simulink model "ICN_with_BR_input_model4test_clusterParams_ParkFig2C_VlungNLR"  (R2020b)
settings: Solver=ode15s  StartTime=0.5  StopTime=480  RelTol=1e-3  EnableMultiTasking=on
model workspace (MAT data in the model file):
  HRResponseIano = [1 0.976355617701 1.05061592575 1.14391807051 1.22959062218 1.30026078221 1.35513299833 1.39551709306 1.423380234 1.44057518669 1.44870724956 1.44945189675 ... (1201 elements, 1x1201)]
values from neighbouring files (symbols this model uses):
  delta_BR = Simulink.Parameter(delta_BR)    [BRclosedLoop_model_initialize_params.m]
  delta_CP = Simulink.Parameter(delta_CP)    [BRclosedLoop_model_initialize_params.m]
  delta_LS = Simulink.Parameter(delta_LS)    [BRclosedLoop_model_initialize_params.m]
  fac0 = 10    [BR_ctrl_params_LBNP_2001.m]    (also in BRmodel_ctrls_LBNP_2001.mat)
  Gal = 23.29    [BR_ctrl_params_LBNP_2001.m]    (also in BRmodel_ctrls_LBNP_2001.mat)
  kBR = Simulink.Parameter(kBR)    [BRclosedLoop_model_initialize_params.m]
  kCP = Simulink.Parameter(kCP)    [BRclosedLoop_model_initialize_params.m]
  kLS = Simulink.Parameter(kLS)    [BRclosedLoop_model_initialize_params.m]
  LBNP_input = Simulink.Parameter(LBNP_input)    [BRclosedLoop_model_initialize_params.m]
  midptCP_gain = Simulink.Parameter(midptCP_gain)    [BRclosedLoop_model_initialize_params.m]
  midptLS_gain = Simulink.Parameter(midptLS_gain)    [BRclosedLoop_model_initialize_params.m]
  minval_BR = Simulink.Parameter(minval_BR)    [BRclosedLoop_model_initialize_params.m]
  minval_CP = Simulink.Parameter(minval_CP)    [BRclosedLoop_model_initialize_params.m]
  minval_LS = Simulink.Parameter(minval_LS)    [BRclosedLoop_model_initialize_params.m]
libraries: simulink x1
(part 2 of 2)

== system ICN_with_BR_input_model4test_clusterParams_ParkFig2C_VlungNLR/Autonomic Nervous System/Emaxlv_inv ==
  fev : Inport
  fes : Inport  Port=2
  Add1 : Sum  Inputs=+++
  Add2 : Sum
  Clock : Clock
  Emaxlv0_denervated (Emaxlv0) : Constant  Value=0.25659999999999994
  Emaxlv_symp : Subsystem
  Emaxlv_vag : Subsystem
  Math Function7 : Math  Operator=reciprocal  SignedPower=on  SaturateOnIntegerOverflow=on
  Pcs_start : Constant
  Scope6 : Scope
  const : Constant  Value=0
  tstall : Switch  Criteria=u2 > Threshold  Threshold=1
  Emaxlv : Outport
  wires:
  Emaxlv_symp/1(1/Emaxlv) -> Scope6/1, Add1/2
  Math Function7/1 -> Add2/1
  Emaxlv_vag/1(1/Emaxlv) -> Add1/1
  Emaxlv0_denervated (Emaxlv0)/1 -> Add2/2
  const/1 -> Add1/3
  Clock/1 -> tstall/2
  Pcs_start/1 -> tstall/3
  tstall/1 -> Math Function7/1
  Add1/1 -> tstall/1
  fes/1 -> Emaxlv_symp/1(fes)
  fev/1 -> Emaxlv_vag/1(fev)
  Add2/1 -> Emaxlv/1

== system ICN_with_BR_input_model4test_clusterParams_ParkFig2C_VlungNLR/Autonomic Nervous System/Emaxrv_inv ==
  fev : Inport
  fes : Inport  Port=2
  Add3 : Sum  Inputs=+++
  Add4 : Sum
  Clock2 : Clock
  Emaxlv0_denervated1 : Constant  Value=1.283*0.5903
  Emaxlv_symp1 : Subsystem
  Emaxlv_vag1 : Subsystem
  Math Function2 : Math  Operator=reciprocal  SignedPower=on  SaturateOnIntegerOverflow=on
  Pcs_start2 : Constant
  Switch2 : Switch  Criteria=u2 > Threshold  Threshold=1
  const1 : Constant  Value=0
  Emaxrv : Outport
  wires:
  Switch2/1 -> Math Function2/1
  Clock2/1 -> Switch2/2
  Add3/1 -> Switch2/1
  Emaxlv_symp1/1(1/Emarlv) -> Add3/2
  Math Function2/1 -> Add4/1
  const1/1 -> Add3/3
  Emaxlv0_denervated1/1 -> Add4/2
  Pcs_start2/1 -> Switch2/3
  Emaxlv_vag1/1(1/Emaxrv) -> Add3/1
  fev/1 -> Emaxlv_vag1/1(fev)
  fes/1 -> Emaxlv_symp1/1(fes)
  Add4/1 -> Emaxrv/1

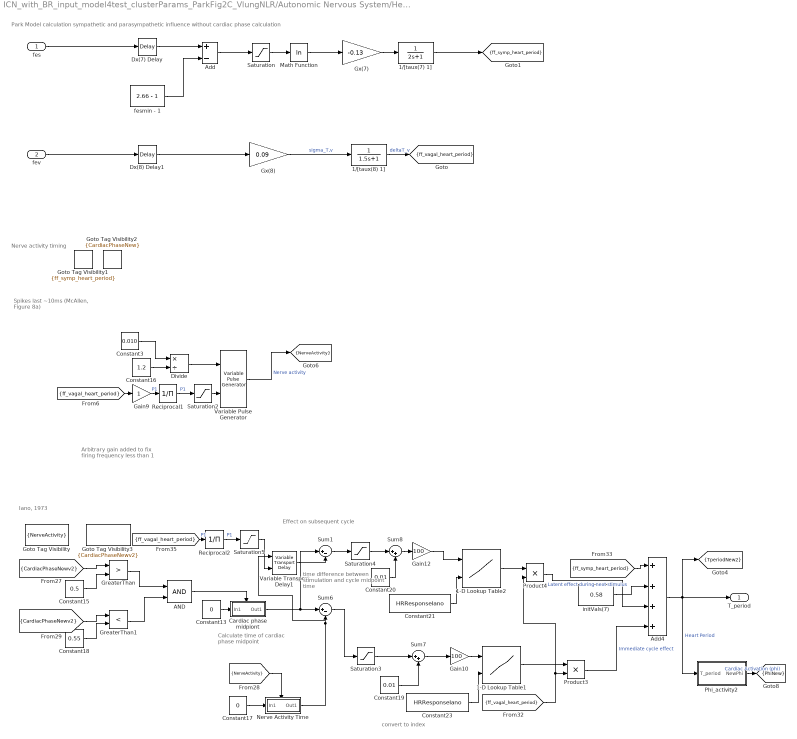
== system ICN_with_BR_input_model4test_clusterParams_ParkFig2C_VlungNLR/Autonomic Nervous System/Heart_period ==
  note: Park Model calculation sympathetic and parasympathetic influence without cardiac phase calculation
  note: Nerve activity timing
  note: convert to index
  note: time difference between stimulation and cycle midpoint time
  note: Calculate time of cardiac phase midpoint
  note: Iano, 1973
  note: Spikes last ~10ms (McAllen, Figure 8a)
  note: Arbitrary gain added to fix firing frequency less than 1
  note: Effect on subsequent cycle
  fes : Inport
  fev : Inport  Port=2
  1-D Lookup Table1 : Lookup_n-D  NumberOfTableDimensions=1  BreakpointsForDimension1=[0:1200]  BreakpointsForDimension2=[0:1199]  TableSource=Input port  Table=tanh([-5:5])  InternalRulePriority=Speed  RndMeth=Simplest  InputSameDT=on
      settings: InputPortMap=u0,p221
  1-D Lookup Table2 : Lookup_n-D  NumberOfTableDimensions=1  BreakpointsForDimension1=[0:1200]  BreakpointsForDimension2=[0:1199]  TableSource=Input port  Table=tanh([-5:5])  InternalRulePriority=Speed  RndMeth=Simplest  InputSameDT=on
      settings: InputPortMap=u0,p221
  1/[taux(7) 1] : TransferFcn  Denominator=[2 1]
  1/[taux(8) 1] : TransferFcn  Denominator=[1.5 1]
  AND : Logic  IconShape=distinctive  AllPortsSameDT=off  OutDataTypeStr=boolean
  Add : Sum  Inputs=+-
  Add4 : Sum  Inputs=++++
  Cardiac phase midpiont : Subsystem  TreatAsAtomicUnit=on
  Constant13 : Constant  Value=0
  Constant15 : Constant  Value=0.5
  Constant16 : Constant  Value=1.2
  Constant17 : Constant  Value=0
  Constant18 : Constant  Value=0.55
  Constant19 : Constant  Value=0.01
  Constant20 : Constant  Value=0.01
  Constant21 : Constant  Value=HRResponseIano
  Constant23 : Constant  Value=HRResponseIano
  Constant3 : Constant  Value=0.010
  Divide : Product  Inputs=*/
  Dx(7) Delay : TransportDelay  DelayTime=2  BufferSize=2048
  Dx(8) Delay1 : TransportDelay  DelayTime=0.2  BufferSize=2048
  Gain10 : Gain  Gain=100
  Gain12 : Gain  Gain=100
  Gain9 : Gain
  Goto Tag Visibility : GotoTagVisibility  GotoTag=NerveActivity
  Goto Tag Visibility1 : GotoTagVisibility  GotoTag=ff_symp_heart_period
  Goto Tag Visibility2 : GotoTagVisibility  GotoTag=CardiacPhaseNew
  Goto Tag Visibility3 : GotoTagVisibility  GotoTag=CardiacPhaseNewv2
  GreaterThan : RelationalOperator  Operator=>  OutDataTypeStr=boolean  RndMeth=Simplest
  GreaterThan1 : RelationalOperator  Operator=<  OutDataTypeStr=boolean  RndMeth=Simplest
  Gx(7) : Gain  Gain=-0.13
  Gx(8) : Gain  Gain=0.09
  Math Function : Math  Operator=log  SignedPower=on  SaturateOnIntegerOverflow=on
  Nerve Activity Time : Subsystem  TreatAsAtomicUnit=on
  Phi_activity2 : Subsystem
  Product3 : Product
  Product4 : Product
  Reciprocal1 : Product  Inputs=/
  Reciprocal2 : Product  Inputs=/
  Saturation : Saturate  UpperLimit=inf  LowerLimit=1
  Saturation2 : Saturate  UpperLimit=10
  Saturation3 : Saturate  UpperLimit=inf  LowerLimit=0
  Saturation4 : Saturate  UpperLimit=inf  LowerLimit=0
  Saturation5 : Saturate  UpperLimit=10
  Sum1 : Sum  Inputs=|+-
  Sum6 : Sum  Inputs=|+-
  Sum7 : Sum  Inputs=|++
  Sum8 : Sum  Inputs=|++
  Variable Transport Delay1 : VariableTransportDelay  VariableDelayType=Variable transport delay  MaximumDelay=10  MaximumPoints=2048
  Variable Pulse Generator : VariablePulseGenerator  AllowZeroPulseWidth=on  SampleTime=0.1
  fesmin - 1 : Constant  Value=2.66 - 1
  initVals(7) : Constant  Value=0.58
  T_period : Outport
  tag scope: NerveActivity=scoped, PhiNew=scoped, TperiodNew2=scoped, ff_symp_heart_period=scoped, ff_vagal_heart_period=scoped
  wires:
  Dx(7) Delay/1 -> Add/1
  fesmin - 1/1 -> Add/2
  Add/1 -> Saturation/1
  Saturation/1 -> Math Function/1
  Math Function/1 -> Gx(7)/1
  Gx(7)/1 -> 1/[taux(7) 1]/1
  fes/1 -> Dx(7) Delay/1
  fev/1 -> Dx(8) Delay1/1
  Dx(8) Delay1/1 -> Gx(8)/1
  Gx(8)/1 -> 1/[taux(8) 1]/1  "sigma_T,v"
  1/[taux(7) 1]/1 -> [ff_symp_heart_period]
  1/[taux(8) 1]/1 -> [ff_vagal_heart_period]  "deltaT_v"
  Constant3/1 -> Divide/1
  Divide/1 -> Variable Pulse Generator/1
  Constant16/1 -> Divide/2
  Variable Pulse Generator/1 -> [NerveActivity]  "Nerve activity"
  Gain9/1 -> Reciprocal1/1  "P1"
  [ff_vagal_heart_period] -> Gain9/1
  Reciprocal1/1 -> Saturation2/1  "P1"
  Saturation2/1 -> Variable Pulse Generator/2
  1-D Lookup Table1/1 -> Product3/1
  Constant13/1 -> Cardiac phase midpiont/1(In1)
  [NerveActivity] -> Nerve Activity Time/Trigger
  Constant17/1 -> Nerve Activity Time/1(In1)
  Nerve Activity Time/1(Out1) -> Variable Transport Delay1/1, Sum6/2
  [CardiacPhaseNewv2] -> GreaterThan/1
  Constant15/1 -> GreaterThan/2
  Constant18/1 -> GreaterThan1/2
  [CardiacPhaseNewv2] -> GreaterThan1/1
  GreaterThan/1 -> AND/1
  GreaterThan1/1 -> AND/2
  AND/1 -> Cardiac phase midpiont/Trigger
  Constant19/1 -> Sum7/2
  Gain10/1 -> 1-D Lookup Table1/1
  Sum7/1 -> Gain10/1
  Saturation3/1 -> Sum7/1
  Sum6/1 -> Saturation3/1
  Add4/1 -> T_period/1, [TperiodNew2], Phi_activity2/1(T_period)  "Heart Period"
  [ff_symp_heart_period] -> Add4/1
  initVals(7)/1 -> Add4/2
  Cardiac phase midpiont/1(Out1) -> Sum1/1, Sum6/1
  Sum1/1 -> Saturation4/1
  Saturation4/1 -> Sum8/1
  Constant20/1 -> Sum8/2
  Sum8/1 -> Gain12/1
  Gain12/1 -> 1-D Lookup Table2/1
  Constant21/1 -> 1-D Lookup Table2/2
  1-D Lookup Table2/1 -> Product4/1
  Product4/1 -> Add4/3  "Latent effect during next stimulus"
  [ff_vagal_heart_period] -> Product4/2, Product3/2
  Variable Transport Delay1/1 -> Sum1/2
  Saturation5/1 -> Variable Transport Delay1/2
  [ff_vagal_heart_period] -> Reciprocal2/1  "P1"
  Reciprocal2/1 -> Saturation5/1  "P1"
  Constant23/1 -> 1-D Lookup Table1/2
  Product3/1 -> Add4/4  "Immediate cycle effect"
  Phi_activity2/1(NewPhi) -> [PhiNew]  "Cardiac Activation (phi)"

== system ICN_with_BR_input_model4test_clusterParams_ParkFig2C_VlungNLR/Autonomic Nervous System/ICN ==
  note: ICN
  note: Scoped Variables
  note: Assumptions
      | Inputs to PN can be modeled as linear combinations (Shinohara, 2012; Magosso, "Theoretical analysis...connection", 2002; Park, 2020)
      | Inputs to LCN can be modeled as linear combinations with sympathetic inputs decreasing firing frequency (negative gain)
      | Only one set of LCNs (same LCN firing frequency goes to the DMV and NA principal neruons)
  fesh : Inport
  fevHR : Inport  Port=2
  fevEmax : Inport  Port=3
  fabr : Inport  Port=4
  Goto Tag Visibility1 : GotoTagVisibility  GotoTag=HR_ICN
  Goto Tag Visibility2 : GotoTagVisibility  GotoTag=phi_ICN
  Goto Tag Visibility3 : GotoTagVisibility  GotoTag=Emaxlv_ICN
  LCN : Subsystem
  PN-DMV : Subsystem
      settings: PortSchema="{\"entries\":[{\"content\":{\"sides\":[{\"content\":{\"connectorIds\":[\"In1\"]},\"type\":\"ConnectorPlacement.EquallySpacedRectSide\",\"uuid\":\"d579c9fc-b45a-4a3f-b69c-1a8b140cd445\"},{\"content\":{\"connectorIds\":[\"Out1\"],\"side\":\"RIGHT\"},\"type\":\"ConnectorPlacement.EquallySpacedRectSide\",\"uuid\":\"0e605ac8-446d-4e1b-b0e5-7b9f562202d0\"},{\"content\":{\"connectorIds\":[\"In2\"],\"side\":\"TOP\"},\"type\":\"ConnectorPlacement.EquallySpacedRectSide\",\"uuid\":\"2307843b-ee9d-4abf-8a00-d07f8ff12bca\"},{\"content\":{\"connectorIds\":[],\"side\":\"HIDDEN\"},\"type\":\"ConnectorPlacement.EquallySpacedRectSide\",\"uuid\":\"4680f609-716a-4cbc-b0ab-b941df6990b7\"}]},\"type\":\"ConnectorPlacement.EquallySpacedConnector\",\"uuid\":\"a97b8c04-f8fb-4ce5-9bdc-b62bd80eb510\"}],\"packageUris\":[\"http://schema.mathworks.com/mf0/Connector/R2020b\"],\"version\":\"1.0\"}"
  PN-NA : Subsystem
      settings: PortSchema="{\"entries\":[{\"content\":{\"sides\":[{\"content\":{\"connectorIds\":[\"In1\"]},\"type\":\"ConnectorPlacement.EquallySpacedRectSide\",\"uuid\":\"d579c9fc-b45a-4a3f-b69c-1a8b140cd445\"},{\"content\":{\"connectorIds\":[\"Out1\"],\"side\":\"RIGHT\"},\"type\":\"ConnectorPlacement.EquallySpacedRectSide\",\"uuid\":\"0e605ac8-446d-4e1b-b0e5-7b9f562202d0\"},{\"content\":{\"connectorIds\":[],\"side\":\"TOP\"},\"type\":\"ConnectorPlacement.EquallySpacedRectSide\",\"uuid\":\"2307843b-ee9d-4abf-8a00-d07f8ff12bca\"},{\"content\":{\"connectorIds\":[\"In2\"],\"side\":\"BOTTOM\"},\"type\":\"ConnectorPlacement.EquallySpacedRectSide\",\"uuid\":\"5095c59b-788d-467d-b9ae-5586250fef9c\"},{\"content\":{\"connectorIds\":[],\"side\":\"HIDDEN\"},\"type\":\"ConnectorPlacement.EquallySpacedRectSide\",\"uuid\":\"4680f609-716a-4cbc-b0ab-b941df6990b7\"}]},\"type\":\"ConnectorPlacement.EquallySpacedConnector\",\"uuid\":\"a97b8c04-f8fb-4ce5-9bdc-b62bd80eb510\"}],\"packageUris\":[\"http://schema.mathworks.com/mf0/Connector/R2020b\"],\"version\":\"1.0\"}"
  Scope : Scope  NumInputPorts=2
  To Workspace1 : ToWorkspace  VariableName=PN_DMV_ff  SampleTime=-1
  To Workspace13 : ToWorkspace  VariableName=PN_NA_ff  SampleTime=-1
  To Workspace2 : ToWorkspace  VariableName=LCN_ff  SampleTime=-1
  kBR_ICN : Gain
  fevHR_ICN : Outport
  fevEmax_ICN : Outport  Port=2
  tag scope: fev_ICN_DMV=scoped
  wires:
  kBR_ICN/1 -> LCN/3(In2)  "Afferent inputs"
  fevEmax/1 -> Scope/1, PN-DMV/1(from DMV), LCN/2(fevEmax)  "DMV output"
  fevHR/1 -> PN-NA/1(fevHR)  "NA output"
  fesh/1 -> LCN/1(fesh)  "fesh"
  PN-DMV/1(x4) -> To Workspace1/1, fevEmax_ICN/1, [fev_ICN_DMV]  "fevEmax_ICN"
  fabr/1 -> kBR_ICN/1
  PN-NA/1(Out1) -> To Workspace13/1, fevHR_ICN/1  "fevHR_ICN"
  LCN/1("from LCN ") -> PN-NA/2("from LCN "), To Workspace2/1, Scope/2, PN-DMV/2("from LCN ")  "LCN Output"

== system ICN_with_BR_input_model4test_clusterParams_ParkFig2C_VlungNLR/Autonomic Nervous System/Left ventricle ==
  Phi : Inport
  Add1 : Sum  Inputs=+-
  Add2 : Sum  Inputs=-+
  Add3 : Sum
  Constant2 : Constant
  Constant4 : Constant
  Math Function : Math  SignedPower=on  SaturateOnIntegerOverflow=on
  P0lv : Constant  Value=0.92999999999999994
  Product : Product  Inputs=3
  Product1 : Product
  Product2 : Product  Inputs=3
  Subsystem : Subsystem
  Vulv : Constant  Value=30.856799999999996
  kElv : Constant  Value=0.01638
  Pmaxlv : Outport
  wires:
  Subsystem/1(Out1) -> Product/3
  [Emaxlv] -> Product/2
  Phi/1 -> Add2/1, Product/1
  Vulv/1 -> Subsystem/1(Vulv)
  [Vlv] -> Product1/1, Subsystem/2(Vlv)
  kElv/1 -> Product1/2
  Product1/1 -> Math Function/1
  Math Function/1 -> Add1/1
  Constant2/1 -> Add1/2
  Add1/1 -> Product2/1
  P0lv/1 -> Product2/2
  Constant4/1 -> Add2/2
  Add2/1 -> Product2/3
  Product/1 -> Add3/1
  Product2/1 -> Add3/2
  Add3/1 -> Pmaxlv/1

== system ICN_with_BR_input_model4test_clusterParams_ParkFig2C_VlungNLR/Autonomic Nervous System/Lung stretch receptors ==
  Vlungs : Inport
  (1)/(tau_lung 1) : TransferFcn  Denominator=[2 1]
  Gal : Gain  Gain=23.29
  falr : Outport
  wires:
  Vlungs/1 -> Gal/1
  (1)/(tau_lung 1)/1 -> falr/1  "fal"
  Gal/1 -> (1)/(tau_lung 1)/1

== system ICN_with_BR_input_model4test_clusterParams_ParkFig2C_VlungNLR/Autonomic Nervous System/Rep ==
  fesp : Inport
  " (1)/([taux(4) 1])" : TransferFcn  Denominator=[6 1]
  Add : Sum  Inputs=+-
  Add1 : Sum
  Constant : Constant  Value=2.66 - 1
  Dx(4) Delay : TransportDelay  DelayTime=2  BufferSize=2048
  Gx(4) : Gain  Gain=0.653
  Math Function : Math  Operator=log  SignedPower=on  SaturateOnIntegerOverflow=on
  Saturation : Saturate  UpperLimit=inf  LowerLimit=1
  initVals(4) : Constant  Value=0.96
  Rep : Outport
  wires:
  fesp/1 -> Dx(4) Delay/1
  Constant/1 -> Add/2
  Add/1 -> Saturation/1
  Saturation/1 -> Math Function/1
  Math Function/1 -> Gx(4)/1
  Gx(4)/1 -> " (1)/([taux(4) 1])"/1
  initVals(4)/1 -> Add1/2
  Add1/1 -> Rep/1
  " (1)/([taux(4) 1])"/1 -> Add1/1
  Dx(4) Delay/1 -> Add/1

== system ICN_with_BR_input_model4test_clusterParams_ParkFig2C_VlungNLR/Autonomic Nervous System/Right ventricle ==
  Phi : Inport
  Add1 : Sum  Inputs=+-
  Add2 : Sum  Inputs=-+
  Add3 : Sum
  Constant2 : Constant
  Constant4 : Constant
  Math Function : Math  SignedPower=on  SaturateOnIntegerOverflow=on
  P0rv : Constant  Value=1.5
  Product : Product  Inputs=3
  Product1 : Product
  Product2 : Product  Inputs=3
  Subsystem : Subsystem
  Vurv : Constant  Value=40.8
  kErv : Constant  Value=0.011
  Pmaxrv : Outport
  wires:
  Subsystem/1(Out1) -> Product/3
  [Emaxrv] -> Product/2
  Phi/1 -> Add2/1, Product/1
  Vurv/1 -> Subsystem/1(Vurv)
  [Vrv] -> Subsystem/2(Vrv), Product1/1
  kErv/1 -> Product1/2
  Product1/1 -> Math Function/1
  Math Function/1 -> Add1/1
  Constant2/1 -> Add1/2
  Add1/1 -> Product2/1
  P0rv/1 -> Product2/2
  Constant4/1 -> Add2/2
  Add2/1 -> Product2/3
  Product/1 -> Add3/1
  Product2/1 -> Add3/2
  Add3/1 -> Pmaxrv/1

== system ICN_with_BR_input_model4test_clusterParams_ParkFig2C_VlungNLR/Autonomic Nervous System/Rmp ==
  fesp : Inport
  " (1)/[taux(9) 1]" : TransferFcn  Denominator=[6 1]
  Add : Sum  Inputs=+-
  Add1 : Sum
  Gx(9) : Gain  Gain=2.81
  Math Function : Math  Operator=log  SignedPower=on  SaturateOnIntegerOverflow=on
  Saturation : Saturate  UpperLimit=inf  LowerLimit=1
  Transport Dx(9) : TransportDelay  DelayTime=2  BufferSize=2048
  fesmin - 1 : Constant  Value=2.66 - 1
  initVals(8) : Constant  Value=4.13
  Rmp : Outport
  wires:
  fesp/1 -> Transport Dx(9)/1
  fesmin - 1/1 -> Add/2
  Add/1 -> Saturation/1
  Saturation/1 -> Math Function/1
  Math Function/1 -> Gx(9)/1
  Gx(9)/1 -> " (1)/[taux(9) 1]"/1
  initVals(8)/1 -> Add1/2
  Add1/1 -> Rmp/1
  " (1)/[taux(9) 1]"/1 -> Add1/1
  Transport Dx(9)/1 -> Add/1

== system ICN_with_BR_input_model4test_clusterParams_ParkFig2C_VlungNLR/Autonomic Nervous System/Rsp ==
  fesp : Inport
  " (1)/([taux(3) 1])" : TransferFcn  Denominator=[6 1]
  Add : Sum  Inputs=+-
  Add1 : Sum
  Dx(3) Delay : TransportDelay  DelayTime=2  BufferSize=2048
  Gx(3) : Gain  Gain=0.695
  Math Function : Math  Operator=log  SignedPower=on  SaturateOnIntegerOverflow=on
  Saturation : Saturate  UpperLimit=inf  LowerLimit=1
  fesmin - 1 : Constant  Value=2.66 - 1
  initVals(3) : Constant  Value=2.49
  Rsp : Outport
  wires:
  fesp/1 -> Dx(3) Delay/1
  fesmin - 1/1 -> Add/2
  Add/1 -> Saturation/1
  Saturation/1 -> Math Function/1
  Math Function/1 -> Gx(3)/1
  Gx(3)/1 -> " (1)/([taux(3) 1])"/1
  initVals(3)/1 -> Add1/2
  Add1/1 -> Rsp/1
  " (1)/([taux(3) 1])"/1 -> Add1/1
  Dx(3) Delay/1 -> Add/1

== system ICN_with_BR_input_model4test_clusterParams_ParkFig2C_VlungNLR/Autonomic Nervous System/Vuev ==
  fev : Inport
  " 1/[taux(6) 1]" : TransferFcn  Denominator=[20 1]
  Add : Sum  Inputs=+-
  Add1 : Sum
  Dx(6) : TransportDelay  DelayTime=5  BufferSize=2048
  Gx(6) : Gain  Gain=-107.5
  Math Function : Math  Operator=log  SignedPower=on  SaturateOnIntegerOverflow=on
  Saturation : Saturate  UpperLimit=inf  LowerLimit=1
  Scope5 : Scope
  fesmin - 1 : Constant  Value=2.66 - 1
  initVals(6) : Constant  Value=1247
  Vuev : Outport
  tag scope: dVuev=scoped
  wires:
  fev/1 -> Dx(6)/1
  fesmin - 1/1 -> Add/2
  Add/1 -> Saturation/1
  Saturation/1 -> Math Function/1
  Math Function/1 -> Gx(6)/1
  Gx(6)/1 -> " 1/[taux(6) 1]"/1
  initVals(6)/1 -> Add1/2
  Add1/1 -> Vuev/1
  " 1/[taux(6) 1]"/1 -> Scope5/1, [dVuev], Add1/1
  Dx(6)/1 -> Add/1

== system ICN_with_BR_input_model4test_clusterParams_ParkFig2C_VlungNLR/Autonomic Nervous System/Vumv ==
  fev : Inport
  " (1)/[taux(10) 1]" : TransferFcn  Denominator=[20 1]
  Add : Sum  Inputs=+-
  Add1 : Sum
  "Dx(10) " : TransportDelay  DelayTime=5  BufferSize=2048
  Gx(10) : Gain  Gain=-25
  Math Function : Math  Operator=log  SignedPower=on  SaturateOnIntegerOverflow=on
  Saturation : Saturate  UpperLimit=inf  LowerLimit=1
  Scope5 : Scope
  fesmin-1 : Constant  Value=2.66 - 1
  initVals(9) : Constant  Value=290
  Vumv : Outport
  tag scope: dVumv=scoped
  wires:
  fev/1 -> "Dx(10) "/1
  fesmin-1/1 -> Add/2
  Add/1 -> Saturation/1
  Saturation/1 -> Math Function/1
  Math Function/1 -> Gx(10)/1
  Gx(10)/1 -> " (1)/[taux(10) 1]"/1
  initVals(9)/1 -> Add1/2
  Add1/1 -> Vumv/1
  " (1)/[taux(10) 1]"/1 -> [dVumv], Scope5/1, Add1/1
  "Dx(10) "/1 -> Add/1

== system ICN_with_BR_input_model4test_clusterParams_ParkFig2C_VlungNLR/Autonomic Nervous System/Vusv ==
  fev : Inport
  " 1/[taux(5) 1]" : TransferFcn  Denominator=[20 1]
  Add : Sum  Inputs=+-
  Add1 : Sum
  Dx(5) Delay : TransportDelay  DelayTime=5  BufferSize=2048
  Gx(5) : Gain  Gain=-265.4
  Math Function : Math  Operator=log  SignedPower=on  SaturateOnIntegerOverflow=on
  Saturation : Saturate  UpperLimit=inf  LowerLimit=1
  fesmin - 1 : Constant  Value=2.66 - 1
  initVals(5) : Constant  Value=1.4354e3
  Vusv : Outport
  wires:
  fev/1 -> Dx(5) Delay/1
  fesmin - 1/1 -> Add/2
  Add/1 -> Saturation/1
  Saturation/1 -> Math Function/1
  Math Function/1 -> Gx(5)/1
  Gx(5)/1 -> " 1/[taux(5) 1]"/1
  initVals(5)/1 -> Add1/2
  Add1/1 -> Vusv/1
  " 1/[taux(5) 1]"/1 -> Add1/1
  Dx(5) Delay/1 -> Add/1

== system ICN_with_BR_input_model4test_clusterParams_ParkFig2C_VlungNLR/Left Heart/Subsystem2 ==
  Pmax : Inport
  P : Inport  Port=2
  Divide : Product  Inputs=/*
  Saturation : Saturate  UpperLimit=inf  LowerLimit=0.01
  kRlv : Gain  Gain=0.00060375
  Fol : Outport
  wires:
  Pmax/1 -> kRlv/1
  P/1 -> Divide/2
  kRlv/1 -> Saturation/1
  Divide/1 -> Fol/1
  Saturation/1 -> Divide/1

== system ICN_with_BR_input_model4test_clusterParams_ParkFig2C_VlungNLR/Right Heart/Subsystem1 ==
  Pmaxrv : Inport
  DP : Inport  Port=2
  Divide : Product  Inputs=/*
  Saturation : Saturate  UpperLimit=inf  LowerLimit=0.01
  kRrv : Gain  Gain=0.0014
  For : Outport
  wires:
  Pmaxrv/1 -> kRrv/1
  DP/1 -> Divide/2
  kRrv/1 -> Saturation/1
  Saturation/1 -> Divide/1
  Divide/1 -> For/1

== system ICN_with_BR_input_model4test_clusterParams_ParkFig2C_VlungNLR/Thoracic Cavity/Thoracic cond. 1 ==
  S (resp) : Inport
  Add : Sum  Inputs=-+
  Add1 : Sum  Inputs=-+
  Divide : Product  Inputs=*/
  Product : Product  Inputs=3
  PthorMax : Constant  Value=-4
  PthorMin : Constant  Value=-9
  Scope : Scope
  Tinsp : Constant  Value=1.6
  Tresp : Constant  Value=4
  Out1 : Outport
  wires:
  Tresp/1 -> Divide/1
  Tinsp/1 -> Divide/2
  Product/1 -> Add1/1
  Add/1 -> Product/3
  Add1/1 -> Scope/1, Out1/1
  S (resp)/1 -> Product/1
  PthorMin/1 -> Add/1
  PthorMax/1 -> Add1/2, Add/2
  Divide/1 -> Product/2

== system ICN_with_BR_input_model4test_clusterParams_ParkFig2C_VlungNLR/Thoracic Cavity/Thoracic cond. 2 ==
  S (resp) : Inport
  Add : Sum  Inputs=-+
  Add1 : Sum  Inputs=-+
  Add2 : Sum  Inputs=-++
  Divide : Product  Inputs=/*
  Product : Product
  Product1 : Product
  PthorMax : Constant  Value=-4
  PthorMin : Constant  Value=-9
  Scope : Scope
  Texp : Constant  Value=1.4
  Tinsp : Constant  Value=1.6
  Tresp : Constant  Value=4
  Out1 : Outport
  wires:
  Tresp/1 -> Product1/2
  Tinsp/1 -> Add2/2
  Product/1 -> Add1/1
  Add1/1 -> Scope/1, Out1/1
  S (resp)/1 -> Product1/1
  PthorMin/1 -> Add/1
  PthorMax/1 -> Add1/2, Add/2
  Texp/1 -> Divide/1, Add2/3
  Product1/1 -> Add2/1
  Add2/1 -> Product/1
  Add/1 -> Divide/2
  Divide/1 -> Product/2

== system ICN_with_BR_input_model4test_clusterParams_ParkFig2C_VlungNLR/Autonomic Nervous System/Brainstem Vagal efferents /NA ==
  fabr : Inport
  Constant1 : Constant
  Divide2 : Product  Inputs=*/
  Divide3 : Product  Inputs=*/
  Exp1 : Math  Operator=pow  SaturateOnIntegerOverflow=on
  NAmidpt : Constant  Commented=on  Value=19.35
  Sum1 : Sum  Inputs=|+-
  Sum3 : Sum  Inputs=|++
  Sum4 : Sum  Inputs=|++
  alpha : Constant  Value=4.875
  beta : Constant  Value=4.875+10.9
  fmidgain : Gain
  "k, gain" : Constant  Value=23
  input : Outport
  tag scope: maxout_NA=scoped
  wires:
  Constant1/1 -> Sum3/1
  fabr/1 -> Divide3/1
  [midPt_NA] -> fmidgain/1
  fmidgain/1 -> Divide3/2
  Divide3/1 -> Exp1/1
  "k, gain"/1 -> Exp1/2
  Exp1/1 -> Sum3/2
  Sum3/1 -> Divide2/2
  Divide2/1 -> Sum4/2
  alpha/1 -> Sum1/1
  beta/1 -> Sum1/2, [maxout_NA], Sum4/1  "beta"
  Sum4/1 -> input/1
  Sum1/1 -> Divide2/1

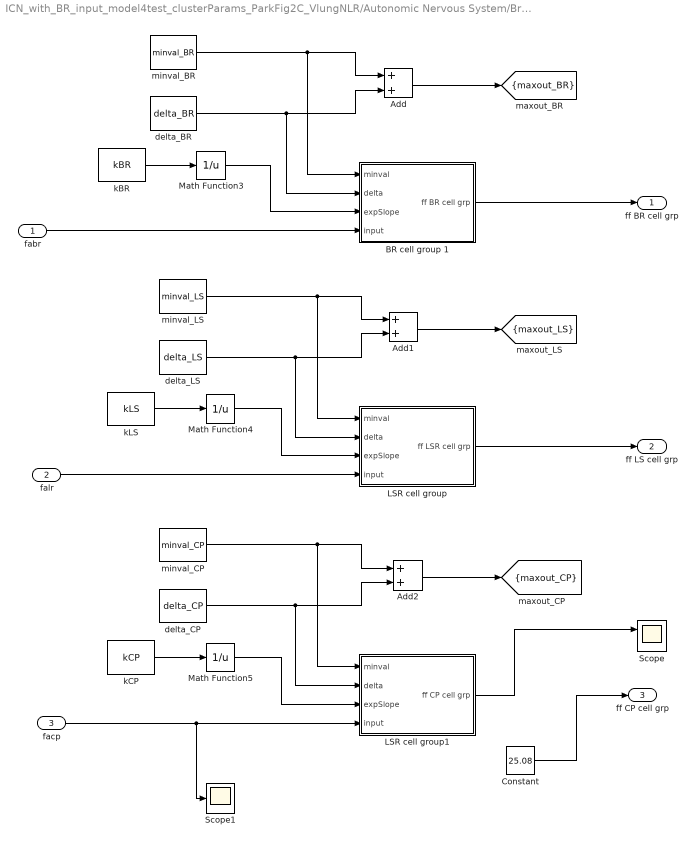
== system ICN_with_BR_input_model4test_clusterParams_ParkFig2C_VlungNLR/Autonomic Nervous System/Brainstem Vagal efferents /NTS1 ==
  fabr : Inport
  falr : Inport  Port=2
  facp : Inport  Port=3
  Add : Sum
  Add1 : Sum
  Add2 : Sum
  BR cell group 1 : Subsystem
  Constant : Constant  Value=25.08
  LSR cell group : Subsystem
  LSR cell group1 : Subsystem
  Math Function3 : Math  Operator=reciprocal  SignedPower=on  SaturateOnIntegerOverflow=on
  Math Function4 : Math  Operator=reciprocal  SignedPower=on  SaturateOnIntegerOverflow=on
  Math Function5 : Math  Operator=reciprocal  SignedPower=on  SaturateOnIntegerOverflow=on
  Scope : Scope  NumInputPorts=2
  Scope1 : Scope
  delta_BR : Constant  Value=delta_BR
  delta_CP : Constant  Value=delta_CP
  delta_LS : Constant  Value=delta_LS
  kBR : Constant  Value=kBR
  kCP : Constant  Value=kCP
  kLS : Constant  Value=kLS
  minval_BR : Constant  Value=minval_BR
  minval_CP : Constant  Value=minval_CP
  minval_LS : Constant  Value=minval_LS
  ff BR cell grp : Outport
  ff LS cell grp : Outport  Port=2
  ff CP cell grp : Outport  Port=3
  tag scope: maxout_BR=scoped, maxout_CP=scoped, maxout_LS=scoped
  wires:
  kBR/1 -> Math Function3/1
  Math Function3/1 -> BR cell group 1/3(expSlope)
  delta_BR/1 -> BR cell group 1/2(delta), Add/2
  fabr/1 -> BR cell group 1/4(input)
  minval_BR/1 -> BR cell group 1/1(minval), Add/1
  kLS/1 -> Math Function4/1
  Math Function4/1 -> LSR cell group/3(expSlope)
  delta_LS/1 -> Add1/2, LSR cell group/2(delta)
  minval_LS/1 -> LSR cell group/1(minval), Add1/1
  LSR cell group/1(ff LSR cell grp) -> ff LS cell grp/1
  BR cell group 1/1(ff BR cell grp) -> ff BR cell grp/1
  falr/1 -> LSR cell group/4(input)
  kCP/1 -> Math Function5/1
  Math Function5/1 -> LSR cell group1/3(expSlope)
  delta_CP/1 -> LSR cell group1/2(delta), Add2/2
  facp/1 -> Scope1/1, LSR cell group1/4(input)
  Add1/1 -> [maxout_LS]
  Add2/1 -> [maxout_CP]
  Add/1 -> [maxout_BR]
  minval_CP/1 -> Add2/1, LSR cell group1/1(minval)
  LSR cell group1/1(ff CP cell grp) -> Scope/1
  Constant/1 -> ff CP cell grp/1

== system ICN_with_BR_input_model4test_clusterParams_ParkFig2C_VlungNLR/Autonomic Nervous System/Brainstem Vagal efferents /New Sigmoid Form2 ==
  input : Inport
  Constant1 : Constant
  Divide2 : Product  Inputs=*/
  Divide3 : Product  Inputs=*/
  Exp1 : Math  Operator=pow  SaturateOnIntegerOverflow=on
  Sum1 : Sum  Inputs=|+-
  Sum3 : Sum  Inputs=|++
  Sum4 : Sum  Inputs=|++
  alpha : Constant  Value=2.5901
  beta : Constant  Value=2.5901+4.0696
  fmidgain : Gain
  fmidinput : Constant  Value=42.91
  "k, gain" : Constant  Value=33.5
  Out1 : Outport
  wires:
  Sum1/1 -> Divide2/1
  Sum4/1 -> Out1/1
  beta/1 -> Sum4/1, Sum1/2  "beta"
  alpha/1 -> Sum1/1
  Divide2/1 -> Sum4/2
  Sum3/1 -> Divide2/2
  Exp1/1 -> Sum3/2
  "k, gain"/1 -> Exp1/2
  Divide3/1 -> Exp1/1
  fmidgain/1 -> Divide3/2
  [midPt_DMV] -> fmidgain/1
  input/1 -> Divide3/1
  Constant1/1 -> Sum3/1

== system ICN_with_BR_input_model4test_clusterParams_ParkFig2C_VlungNLR/Autonomic Nervous System/Brainstem Vagal efferents /New Sigmoid Form3 ==
  input : Inport
  midpt : Inport  Port=2
  Constant1 : Constant
  Divide2 : Product  Inputs=*/
  Divide3 : Product  Inputs=*/
  Exp1 : Math  Operator=pow  SaturateOnIntegerOverflow=on
  Sum1 : Sum  Inputs=|+-
  Sum3 : Sum  Inputs=|++
  Sum4 : Sum  Inputs=|++
  Terminator : Terminator
  alpha : Constant  Value=0.61
  beta : Constant  Value=0.61+10.3919
  fmidgain : Gain
  fmidinput : Constant  Value=9.7805
  "k, gain" : Constant  Value=7
  Out1 : Outport
  wires:
  Constant1/1 -> Sum3/1
  input/1 -> Divide3/1
  fmidinput/1 -> fmidgain/1
  Divide3/1 -> Exp1/1
  "k, gain"/1 -> Exp1/2
  Exp1/1 -> Sum3/2
  Sum3/1 -> Divide2/2
  Divide2/1 -> Sum4/2
  alpha/1 -> Sum1/1
  beta/1 -> Sum1/2, Sum4/1  "beta"
  Sum4/1 -> Out1/1
  Sum1/1 -> Divide2/1
  midpt/1 -> Divide3/2
  fmidgain/1 -> Terminator/1

== system ICN_with_BR_input_model4test_clusterParams_ParkFig2C_VlungNLR/Autonomic Nervous System/Brainstem Vagal efferents /Subsystem2 ==
  Add2 : Sum  Inputs=+++
  Constant : Constant  Value=0.4754+30.2142
  Gain : Gain  Gain=0.5272
  midpt_DMV : Outport
  wires:
  Constant/1 -> Add2/3
  [maxout_BR] -> Add2/1
  Gain/1 -> midpt_DMV/1
  Add2/1 -> Gain/1
  [maxout_LS] -> Add2/2

== system ICN_with_BR_input_model4test_clusterParams_ParkFig2C_VlungNLR/Autonomic Nervous System/Brainstem Vagal efferents /Subsystem3 ==
  Add2 : Sum  Inputs=+++
  Constant : Constant  Value=0.4754+30.2142
  Gain1 : Gain  Gain=0.735
  midpt_NA : Outport
  tag scope: midPt_NA=scoped
  wires:
  Constant/1 -> Add2/3
  [maxout_BR] -> Add2/1
  [maxout_LS] -> Add2/2
  Add2/1 -> Gain1/1
  Gain1/1 -> [midPt_NA], midpt_NA/1

== system ICN_with_BR_input_model4test_clusterParams_ParkFig2C_VlungNLR/Autonomic Nervous System/Emaxlv_inv/Emaxlv_symp ==
  fes : Inport
  (1)/(taux(2) 1) : TransferFcn  Denominator=[8 1]
  Add : Sum  Inputs=+-
  Gain2 : Gain  Gain=-1
  Gs_Emaxlv : Gain  Gain=0.13
  Math Function : Math  Operator=log  SignedPower=on  SaturateOnIntegerOverflow=on
  Saturation : Saturate  UpperLimit=inf  LowerLimit=1
  Transport Dx(1) : TransportDelay  DelayTime=2  BufferSize=2048
  fesmin - 1 : Constant  Value=2.66 - 1
  1/Emaxlv : Outport
  wires:
  fes/1 -> Transport Dx(1)/1
  Transport Dx(1)/1 -> Add/1
  Add/1 -> Saturation/1
  Saturation/1 -> Math Function/1
  Math Function/1 -> Gs_Emaxlv/1
  (1)/(taux(2) 1)/1 -> 1/Emaxlv/1
  fesmin - 1/1 -> Add/2
  Gs_Emaxlv/1 -> Gain2/1
  Gain2/1 -> (1)/(taux(2) 1)/1

== system ICN_with_BR_input_model4test_clusterParams_ParkFig2C_VlungNLR/Autonomic Nervous System/Emaxlv_inv/Emaxlv_vag ==
  fev : Inport
  Gv_Emaxlv : Gain  Gain=0.2053
  To Workspace9 : ToWorkspace  Commented=on  VariableName=fev_Einput  SaveFormat=Timeseries  SampleTime=-1
  Transfer Fcn : TransferFcn  Denominator=[1.5 1]
  Transport Delay : TransportDelay  DelayTime=0.2  BufferSize=2048
  1/Emaxlv : Outport
  wires:
  fev/1 -> Transport Delay/1
  Transport Delay/1 -> To Workspace9/1, Gv_Emaxlv/1
  Transfer Fcn/1 -> 1/Emaxlv/1
  Gv_Emaxlv/1 -> Transfer Fcn/1

== system ICN_with_BR_input_model4test_clusterParams_ParkFig2C_VlungNLR/Autonomic Nervous System/Emaxrv_inv/Emaxlv_symp1 ==
  note: 1/0.5903 gain factor is to account for differences between LV and RV performance
      | (Ursino 1998 model uses a 0.59 factor to account for lower elasticity of RV to LV) - use
      | 1/0.5903 to account for inverse relationship being calculated in this model, which
      | accounts for accentuated antagonism of sympathetic and vagal influences on elasticity
  fes : Inport
  Add : Sum  Inputs=+-
  Constant : Constant  Value=2.66 - 1
  Gain1 : Gain  Gain=0.13
  Gain2 : Gain  Gain=-1
  Gain3 : Gain  Gain=1/0.5903
  Math Function : Math  Operator=log  SignedPower=on  SaturateOnIntegerOverflow=on
  Saturation : Saturate  UpperLimit=inf  LowerLimit=1
  Transfer Fcn : TransferFcn  Denominator=[8 1]
  Transport Delay : TransportDelay  DelayTime=2  BufferSize=2048
  1/Emarlv : Outport
  wires:
  fes/1 -> Transport Delay/1
  Transport Delay/1 -> Add/1
  Add/1 -> Saturation/1
  Saturation/1 -> Math Function/1
  Math Function/1 -> Gain1/1
  Transfer Fcn/1 -> Gain3/1
  Constant/1 -> Add/2
  Gain1/1 -> Gain2/1
  Gain2/1 -> Transfer Fcn/1
  Gain3/1 -> 1/Emarlv/1

== system ICN_with_BR_input_model4test_clusterParams_ParkFig2C_VlungNLR/Autonomic Nervous System/Emaxrv_inv/Emaxlv_vag1 ==
  note: 1/0.5903 gain factor is to account for differences between LV and RV performance
      | (Ursino 1998 model uses a 0.59 factor to account for lower elasticity of RV to LV) - use
      | 1/0.5903 to account for inverse relationship being calculated in this model, which
      | accounts for accentuated antagonism of sympathetic and vagal influences on elasticity
  fev : Inport
  Gain : Gain  Gain=0.2053
  Gain1 : Gain  Gain=1/0.5903
  Transfer Fcn : TransferFcn  Denominator=[1.5 1]
  Transport Delay : TransportDelay  DelayTime=0.2  BufferSize=2048
  1/Emaxrv : Outport
  wires:
  fev/1 -> Transport Delay/1
  Transport Delay/1 -> Gain/1
  Transfer Fcn/1 -> Gain1/1
  Gain/1 -> Transfer Fcn/1
  Gain1/1 -> 1/Emaxrv/1

== system ICN_with_BR_input_model4test_clusterParams_ParkFig2C_VlungNLR/Autonomic Nervous System/Heart_period/Cardiac phase midpiont ==
  In1 : Inport
  Trigger : TriggerPort  TriggerType=either  VariantControl=Variant
  Digital Clock : DigitalClock  SampleTime=-1
  Terminator : Terminator
  Out1 : Outport
  wires:
  Digital Clock/1 -> Out1/1
  In1/1 -> Terminator/1

== system ICN_with_BR_input_model4test_clusterParams_ParkFig2C_VlungNLR/Autonomic Nervous System/Heart_period/Nerve Activity Time ==
  In1 : Inport
  Trigger : TriggerPort  TriggerType=either  VariantControl=Variant
  Digital Clock : DigitalClock  SampleTime=-1
  Terminator : Terminator
  Out1 : Outport
  wires:
  In1/1 -> Terminator/1
  Digital Clock/1 -> Out1/1

== system ICN_with_BR_input_model4test_clusterParams_ParkFig2C_VlungNLR/Autonomic Nervous System/Heart_period/Phi_activity2 ==
  note: u(t)
  note: u(t)
  note: 1/T
  note: Tsys
  note: 1/T
  note: Tsys/T
  note: u*T/Tsys
  T_period : Inport
  Add : Sum  Inputs=-+
  Constant : Constant
  Constant4 : Constant  Value=0
  Divide : Product  Inputs=*/
  Fcn : Fcn  Expr=sin(pi*u(1))^2
  Integrator : Integrator  ExternalReset=falling  ShowStatePort=on
  Math Function : Math  Operator=reciprocal  SignedPower=on  SaturateOnIntegerOverflow=on
  Product : Product
  Product1 : Product
  Sum : Sum  Inputs=-+
  Switch : Switch  Threshold=1
  To Workspace1 : ToWorkspace  Commented=on  VariableName=CardiacPhase  SampleTime=-1
  Tsys0 : Constant  Value=0.4
  ksys : Constant  Value=0.075
  NewPhi : Outport
  tag scope: CardiacPhaseNewv2=scoped
  wires:
  Integrator/1 -> Divide/1, [CardiacPhaseNewv2], To Workspace1/1
  Fcn/1 -> NewPhi/1
  Switch/1 -> Fcn/1
  T_period/1 -> Math Function/1
  Divide/1 -> Switch/2, Switch/3
  Constant4/1 -> Switch/1
  Product1/1 -> Divide/2
  Add/1 -> Product1/2
  Tsys0/1 -> Add/2
  Product/1 -> Add/1
  ksys/1 -> Product/2
  Math Function/1 -> Integrator/1, Product1/1, Product/1
  Sum/1 -> Integrator/2
  Constant/1 -> Sum/2
  Integrator/State -> Sum/1

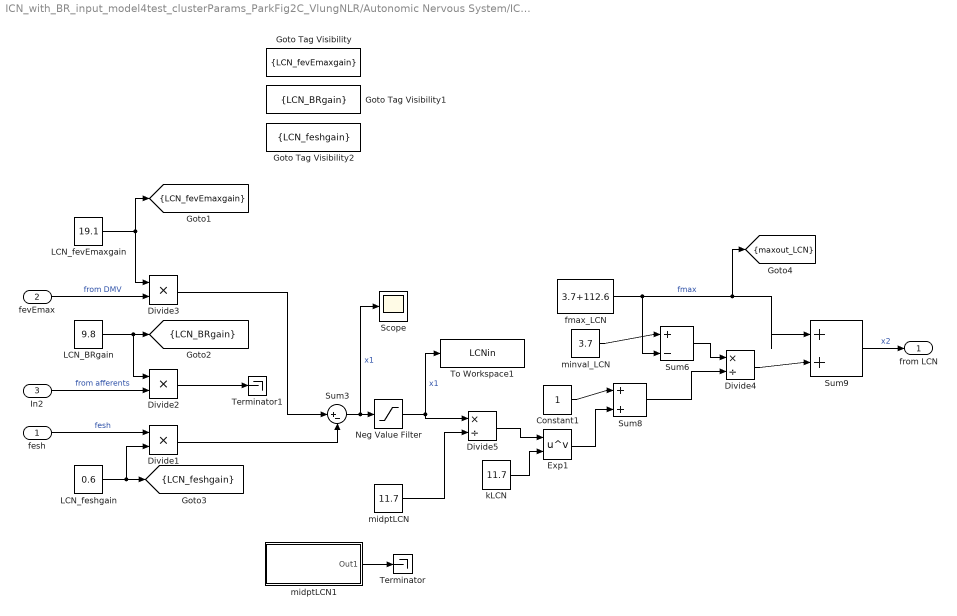
== system ICN_with_BR_input_model4test_clusterParams_ParkFig2C_VlungNLR/Autonomic Nervous System/ICN/LCN ==
  fesh : Inport
  fevEmax : Inport  Port=2
  In2 : Inport  Port=3
  Constant1 : Constant
  Divide1 : Product  Inputs=**
  Divide2 : Product  Inputs=**
  Divide3 : Product  Inputs=**
  Divide4 : Product  Inputs=*/
  Divide5 : Product  Inputs=*/
  Exp1 : Math  Operator=pow  SaturateOnIntegerOverflow=on
  Goto Tag Visibility : GotoTagVisibility  GotoTag=LCN_fevEmaxgain
  Goto Tag Visibility1 : GotoTagVisibility  GotoTag=LCN_BRgain
  Goto Tag Visibility2 : GotoTagVisibility  GotoTag=LCN_feshgain
  LCN_BRgain : Constant  Value=9.8
  LCN_feshgain : Constant  Value=0.6
  LCN_fevEmaxgain : Constant  Value=19.1
  Neg Value Filter : Saturate  UpperLimit=inf  LowerLimit=0
  Scope : Scope
  Sum3 : Sum  Inputs=|+-
  Sum6 : Sum  Inputs=|+-
  Sum8 : Sum  Inputs=|++
  Sum9 : Sum  Inputs=|++
  Terminator : Terminator
  Terminator1 : Terminator
  To Workspace1 : ToWorkspace  VariableName=LCNin  SampleTime=-1
  fmax_LCN : Constant  Value=3.7+112.6
  kLCN : Constant  Value=11.7
  midptLCN : Constant  Value=11.7
  midptLCN1 : Subsystem
  minval_LCN : Constant  Value=3.7
  "from LCN " : Outport
  tag scope: LCN_BRgain=scoped, LCN_feshgain=scoped, LCN_fevEmaxgain=scoped, maxout_LCN=scoped
  wires:
  fevEmax/1 -> Divide3/2  "from DMV"
  Divide2/1 -> Terminator1/1
  In2/1 -> Divide2/2  "from afferents"
  Divide3/1 -> Sum3/1
  fesh/1 -> Divide1/1  "fesh"
  LCN_feshgain/1 -> Divide1/2, [LCN_feshgain]
  LCN_fevEmaxgain/1 -> [LCN_fevEmaxgain], Divide3/1
  LCN_BRgain/1 -> [LCN_BRgain], Divide2/1
  Sum3/1 -> Scope/1, Neg Value Filter/1  "x1"
  Exp1/1 -> Sum8/2
  fmax_LCN/1 -> Sum6/2, [maxout_LCN], Sum9/1  "fmax"
  Neg Value Filter/1 -> To Workspace1/1, Divide5/1  "x1"
  Sum6/1 -> Divide4/1
  kLCN/1 -> Exp1/2
  Divide4/1 -> Sum9/2
  Sum8/1 -> Divide4/2
  Constant1/1 -> Sum8/1
  minval_LCN/1 -> Sum6/1
  midptLCN/1 -> Divide5/2
  Divide5/1 -> Exp1/1
  Sum9/1 -> "from LCN "/1  "x2"
  midptLCN1/1(Out1) -> Terminator/1
  Divide1/1 -> Sum3/2

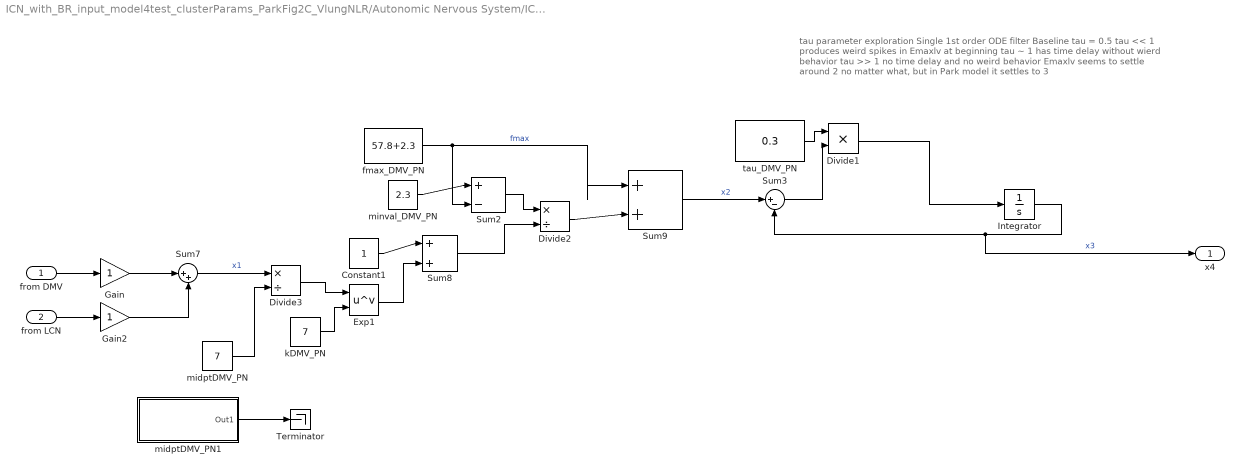
== system ICN_with_BR_input_model4test_clusterParams_ParkFig2C_VlungNLR/Autonomic Nervous System/ICN/PN-DMV ==
  note: tau parameter exploration
      | Single 1st order ODE filter
      | Baseline tau = 0.5
      | tau << 1 produces weird spikes in Emaxlv at beginning
      | tau ~ 1 has time delay without wierd behavior
      | tau >> 1 no time delay and no weird behavior
      | Emaxlv seems to settle around 2 no matter what, but in Park model it settles to 3
  from DMV : Inport
  "from LCN " : Inport  Port=2
  Constant1 : Constant
  Divide1 : Product  Inputs=**
  Divide2 : Product  Inputs=*/
  Divide3 : Product  Inputs=*/
  Exp1 : Math  Operator=pow  SaturateOnIntegerOverflow=on
  Gain : Gain
  Gain2 : Gain
  Integrator : Integrator
  Sum2 : Sum  Inputs=|+-
  Sum3 : Sum  Inputs=|+-
  Sum7 : Sum  Inputs=|++
  Sum8 : Sum  Inputs=|++
  Sum9 : Sum  Inputs=|++
  Terminator : Terminator
  fmax_DMV_PN : Constant  Value=57.8+2.3
  kDMV_PN : Constant  Value=7
  midptDMV_PN : Constant  Value=7
  midptDMV_PN1 : Subsystem
  minval_DMV_PN : Constant  Value=2.3
  tau_DMV_PN : Constant  Value=0.3
  x4 : Outport
  wires:
  from DMV/1 -> Gain/1
  "from LCN "/1 -> Gain2/1
  Sum3/1 -> Divide1/2
  Integrator/1 -> x4/1, Sum3/2  "x3"
  Sum9/1 -> Sum3/1  "x2"
  Divide1/1 -> Integrator/1
  tau_DMV_PN/1 -> Divide1/1
  Exp1/1 -> Sum8/2
  fmax_DMV_PN/1 -> Sum2/2, Sum9/1  "fmax"
  Sum2/1 -> Divide2/1
  kDMV_PN/1 -> Exp1/2
  Divide3/1 -> Exp1/1
  minval_DMV_PN/1 -> Sum2/1
  Gain2/1 -> Sum7/2
  Gain/1 -> Sum7/1
  Constant1/1 -> Sum8/1
  Sum8/1 -> Divide2/2
  midptDMV_PN/1 -> Divide3/2
  Divide2/1 -> Sum9/2
  midptDMV_PN1/1(Out1) -> Terminator/1
  Sum7/1 -> Divide3/1  "x1"

== system ICN_with_BR_input_model4test_clusterParams_ParkFig2C_VlungNLR/Autonomic Nervous System/ICN/PN-NA ==
  fevHR : Inport
  "from LCN " : Inport  Port=2
  Constant1 : Constant
  Divide2 : Product  Inputs=*/
  Divide3 : Product  Inputs=*/
  Exp1 : Math  Operator=pow  SaturateOnIntegerOverflow=on
  Gain : Gain
  Gain2 : Gain
  Sum2 : Sum  Inputs=|+-
  Sum4 : Sum  Inputs=|++
  Sum6 : Sum  Inputs=|++
  Sum7 : Sum  Inputs=|++
  Terminator : Terminator
  Transport Delay1 : TransportDelay  Commented=on  DelayTime=0.1
  fmax_NA_PN : Constant  Value=48.8+2.7
  kNA : Constant  Value=7
  midptNA_PN : Constant  Value=7
  midptNA_PN1 : Subsystem
  minval_NA_PN : Constant  Value=2.7
  Out1 : Outport
  wires:
  Gain/1 -> Sum4/1
  "from LCN "/1 -> Gain2/1  "from LCN"
  fevHR/1 -> Gain/1  "from NA"
  Gain2/1 -> Sum4/2
  minval_NA_PN/1 -> Sum2/1
  kNA/1 -> Exp1/2
  Sum2/1 -> Divide2/1
  Sum7/1 -> Out1/1
  fmax_NA_PN/1 -> Sum2/2, Sum7/1  "fmax"
  Sum6/1 -> Divide2/2
  Constant1/1 -> Sum6/1
  Divide3/1 -> Exp1/1
  Divide2/1 -> Sum7/2
  Exp1/1 -> Sum6/2
  midptNA_PN/1 -> Divide3/2
  midptNA_PN1/1(Out1) -> Terminator/1
  Sum4/1 -> Divide3/1  "x1"

== system ICN_with_BR_input_model4test_clusterParams_ParkFig2C_VlungNLR/Autonomic Nervous System/Left ventricle/Subsystem ==
  Vulv : Inport
  Vlv : Inport  Port=2
  Add : Sum  Inputs=-+
  Saturation : Saturate  UpperLimit=10000  LowerLimit=0
  Out1 : Outport
  wires:
  Vulv/1 -> Add/1
  Vlv/1 -> Add/2
  Add/1 -> Saturation/1
  Saturation/1 -> Out1/1

== system ICN_with_BR_input_model4test_clusterParams_ParkFig2C_VlungNLR/Autonomic Nervous System/Right ventricle/Subsystem ==
  Vurv : Inport
  Vrv : Inport  Port=2
  Add : Sum  Inputs=-+
  Saturation : Saturate  UpperLimit=10000  LowerLimit=0
  Out1 : Outport
  wires:
  Vurv/1 -> Add/1
  Vrv/1 -> Add/2
  Add/1 -> Saturation/1
  Saturation/1 -> Out1/1

== system ICN_with_BR_input_model4test_clusterParams_ParkFig2C_VlungNLR/Autonomic Nervous System/Brainstem Vagal efferents /NTS1/BR cell group 1 ==
  minval : Inport
  delta : Inport  Port=2
  expSlope : Inport  Port=3
  input : Inport  Port=4
  Add1 : Sum
  Add2 : Sum
  Add3 : Sum  Inputs=-+
  Add4 : Sum
  BR mid-point : Constant  Value=25
  Constant3 : Constant
  Divide : Product  Inputs=*/
  Gain : Gain  Gain=1.7649
  Math Function2 : Math  SignedPower=on  SaturateOnIntegerOverflow=on
  Product : Product
  Product1 : Product
  ff BR cell grp : Outport
  wires:
  Add2/1 -> Divide/2
  Constant3/1 -> Add2/2
  Math Function2/1 -> Add2/1, Product1/2
  Divide/1 -> ff BR cell grp/1
  Product/1 -> Math Function2/1
  Add3/1 -> Product/1
  expSlope/1 -> Product/2
  input/1 -> Add3/2
  BR mid-point/1 -> Gain/1
  Add1/1 -> Product1/1
  minval/1 -> Add4/1, Add1/1
  delta/1 -> Add1/2
  Product1/1 -> Add4/2
  Add4/1 -> Divide/1
  Gain/1 -> Add3/1

== system ICN_with_BR_input_model4test_clusterParams_ParkFig2C_VlungNLR/Autonomic Nervous System/Brainstem Vagal efferents /NTS1/LSR cell group ==
  minval : Inport
  delta : Inport  Port=2
  expSlope : Inport  Port=3
  input : Inport  Port=4
  Add1 : Sum
  Add2 : Sum
  Add3 : Sum  Inputs=-+
  Add4 : Sum
  Constant3 : Constant
  Divide : Product  Inputs=*/
  Gain : Gain  Gain=midptLS_gain
  LSR mid-point : Constant  Value=Gal/2
  Math Function2 : Math  SignedPower=on  SaturateOnIntegerOverflow=on
  Product : Product
  Product1 : Product
  ff LSR cell grp : Outport
  wires:
  Add2/1 -> Divide/2
  Constant3/1 -> Add2/2
  Math Function2/1 -> Add2/1, Product1/2
  Divide/1 -> ff LSR cell grp/1
  Product/1 -> Math Function2/1
  Add3/1 -> Product/1
  expSlope/1 -> Product/2
  input/1 -> Add3/2
  LSR mid-point/1 -> Gain/1
  Add1/1 -> Product1/1
  minval/1 -> Add4/1, Add1/1
  delta/1 -> Add1/2
  Product1/1 -> Add4/2
  Add4/1 -> Divide/1
  Gain/1 -> Add3/1

== system ICN_with_BR_input_model4test_clusterParams_ParkFig2C_VlungNLR/Autonomic Nervous System/Brainstem Vagal efferents /NTS1/LSR cell group1 ==
  minval : Inport
  delta : Inport  Port=2
  expSlope : Inport  Port=3
  input : Inport  Port=4
  Add1 : Sum
  Add2 : Sum
  Add3 : Sum  Inputs=-+
  Add4 : Sum
  CP mid-point : Constant  Value=fac0
  Constant3 : Constant
  Divide : Product  Inputs=*/
  Gain : Gain  Gain=midptCP_gain
  Math Function2 : Math  SignedPower=on  SaturateOnIntegerOverflow=on
  Product : Product
  Product1 : Product
  ff CP cell grp : Outport
  wires:
  Add2/1 -> Divide/2
  Constant3/1 -> Add2/2
  Math Function2/1 -> Add2/1, Product1/2
  Divide/1 -> ff CP cell grp/1
  Product/1 -> Math Function2/1
  Add3/1 -> Product/1
  expSlope/1 -> Product/2
  input/1 -> Add3/2
  CP mid-point/1 -> Gain/1
  Add1/1 -> Product1/1
  minval/1 -> Add4/1, Add1/1
  delta/1 -> Add1/2
  Product1/1 -> Add4/2
  Add4/1 -> Divide/1
  Gain/1 -> Add3/1

== system ICN_with_BR_input_model4test_clusterParams_ParkFig2C_VlungNLR/Autonomic Nervous System/ICN/LCN/midptLCN1 ==
  Divide{,1..2,4} (4 alike) : Product  Inputs=**
  Sum : Sum  Inputs=|+++
  midptLCN_gain : Constant  Value=4.7
  Out1 : Outport
  wires:
  Divide/1 -> Out1/1
  [maxout_fevEmax] -> Divide1/1
  Sum/1 -> Divide/2
  midptLCN_gain/1 -> Divide/1
  Divide1/1 -> Sum/1
  [LCN_fevEmaxgain] -> Divide1/2
  [maxout_fabr] -> Divide2/1
  [LCN_BRgain] -> Divide2/2
  Divide2/1 -> Sum/2
  [fesh] -> Divide4/1
  [LCN_feshgain] -> Divide4/2
  Divide4/1 -> Sum/3

== system ICN_with_BR_input_model4test_clusterParams_ParkFig2C_VlungNLR/Autonomic Nervous System/ICN/PN-DMV/midptDMV_PN1 ==
  Divide : Product  Inputs=**
  Sum : Sum  Inputs=|++
  midptDMV_PN_gain : Constant  Value=0.7
  Out1 : Outport
  wires:
  Divide/1 -> Out1/1
  [maxout_LCN] -> Sum/1
  [maxout_fevEmax] -> Sum/2
  Sum/1 -> Divide/2
  midptDMV_PN_gain/1 -> Divide/1

== system ICN_with_BR_input_model4test_clusterParams_ParkFig2C_VlungNLR/Autonomic Nervous System/ICN/PN-NA/midptNA_PN1 ==
  Divide : Product  Inputs=**
  Scope : Scope
  Sum : Sum  Inputs=|++
  midptNA_PN_gain : Constant
  Out1 : Outport
  wires:
  midptNA_PN_gain/1 -> Divide/1
  Sum/1 -> Divide/2
  [maxout_fevHR] -> Scope/1, Sum/2
  [maxout_LCN] -> Sum/1
  Divide/1 -> Out1/1
